simulink model "wushuadianji"  (R2020a)
settings: Solver=FixedStepAuto  StartTime=0.0  StopTime=Inf  FixedStep=Ts  RelTol=1e-3  EnableMultiTasking=on
model workspace (MAT data in the model file):
  Ts = 0.001
libraries: canmsglib x8, speedgoatlib_IO602_4 x3, CanManageLib x3
settings Model: Creator=HIL  LastModifiedBy=HIL
settings SolverCC: ConcurrentTasks=on  AutoInsertRateTranBlk=on
settings DataIOCC: SaveFormat=StructureWithTime
settings OptimizationCC: BlockReduction=off  OptimizeBlockIOStorage=off
settings HardwareCC: ProdBitPerPointer=32  ProdBitPerSizeT=32  ProdBitPerPtrDiffT=32  ProdLargestAtomicFloat=None  ProdWordSize=32  ProdLongLongMode=on  ProdHWDeviceType=Generic->32-bit x86 compatible
settings RTWCC: Description=Simulink Real-Time  SystemTargetFile=slrt.tlc  TemplateMakefile=slrt_default_tmf  CodeExecutionProfiling=on  RTWCompilerOptimization=on
settings SimulinkRealTimeCC: SupportVariableSizeSignals=on  RL32LogTETModifier=off  xPCConcurrentTasks=on

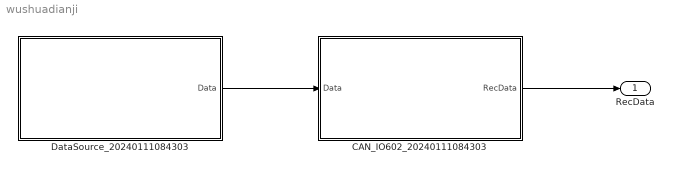
== system wushuadianji ==
  CAN_IO602_20240111084303 : Subsystem
  DataSource_20240111084303 : Subsystem
  RecData : Outport
  wires:
  DataSource_20240111084303/1(Data) -> CAN_IO602_20240111084303/1(Data)
  CAN_IO602_20240111084303/1(RecData) -> RecData/1

== system wushuadianji/CAN_IO602_20240111084303 ==
  Data : Inport
  CAN Receive : Subsystem  TreatAsAtomicUnit=on
  CAN Setup : speedgoatlib_IO602_4/Legacy/CAN Setup   moduletype=IO602  id=1  pciSlot=-1  chn1=CAN (HS)  chn2=CAN (HS)  chn3=Disabled  chn4=Disabled  initStruct=[]  termStruct=[]  ArbitrationbdrChn1=500 kBaud  ArbitrationManbdrChn1=[2,16,63,16]  FdbdrChn1=5.0 MBaud  FdManbdrChn1=[2,2,5,2]  ArbitrationbdrChn2=500 kBaud  ArbitrationManbdrChn2=[2,16,63,16]  FdbdrChn2=5.0 MBaud  FdManbdrChn2=[2,2,5,2]  ArbitrationbdrChn3=1.0 MBaud  ArbitrationManbdrChn3=[2,8,31,8]  FdbdrChn3=5.0 MBaud  FdManbdrChn3=[2,2,5,2]  ArbitrationbdrChn4=1.0 MBaud  ArbitrationManbdrChn4=[2,8,31,8]  FdbdrChn4=5.0 MBaud  FdManbdrChn4=[2,2,5,2]  moduleInitValues=[602 1 -1 -1]
      settings: SourceProductName=Simulink Real-Time: Speedgoat I/O Blockset
  CAN Transmit : Subsystem  TreatAsAtomicUnit=on
  Enable : BusSelector  OutputSignals=Trigger.Enable_CanTransmit
  RecData : Outport
  wires:
  Enable/1 -> CAN Transmit/Enable  "<Enable_CanTransmit>"
  Data/1 -> CAN Transmit/1(Data), Enable/1
  CAN Receive/1(RecData) -> RecData/1

== system wushuadianji/DataSource_20240111084303 ==
  Bus Creator : BusCreator  Inputs=2
  Signal : Subsystem
  Trigger : Subsystem
  Data : Outport
  wires:
  Trigger/1(Trigger) -> Bus Creator/1  "Trigger"
  Signal/1(Signal) -> Bus Creator/2  "Signal"
  Bus Creator/1 -> Data/1  "Data"

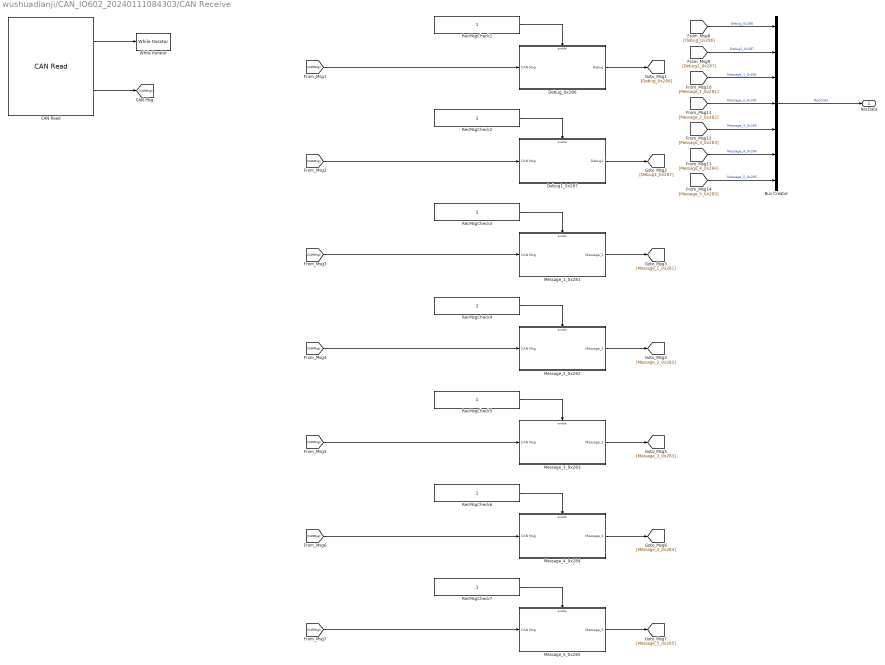
== system wushuadianji/CAN_IO602_20240111084303/CAN Receive ==
  Bus Creator : BusCreator  Inputs=7
  CAN Read : speedgoatlib_IO602_4/Legacy/CAN Read  id=1  ts=-1  channel=1  messageType=CAN  canType=CAN (HS)  BusOutput=on  initValues=[602 1 -1 0 1 1 1]
      settings: SourceProductName=Simulink Real-Time: Speedgoat I/O Blockset
  Debug1_0x287 : Subsystem  TreatAsAtomicUnit=on
  Debug_0x286 : Subsystem  TreatAsAtomicUnit=on
  Message_1_0x281 : Subsystem  TreatAsAtomicUnit=on
  Message_2_0x282 : Subsystem  TreatAsAtomicUnit=on
  Message_3_0x283 : Subsystem  TreatAsAtomicUnit=on
  Message_4_0x284 : Subsystem  TreatAsAtomicUnit=on
  Message_5_0x285 : Subsystem  TreatAsAtomicUnit=on
  RecMsgCheck{1..7} (7 alike) : Constant  OutDataTypeStr=boolean
  While Iterator : WhileIterator  MaxIters=500  WhileBlockType=do-while
  RecData : Outport
  wires:
  CAN Read/1 -> While Iterator/1
  CAN Read/2 -> [CANMsg]
  RecMsgCheck1/1 -> Debug_0x286/Enable
  [CANMsg] -> Debug_0x286/1(CAN Msg)
  Debug_0x286/1(Debug) -> [Debug_0x286]
  RecMsgCheck2/1 -> Debug1_0x287/Enable
  [CANMsg] -> Debug1_0x287/1(CAN Msg)
  Debug1_0x287/1(Debug1) -> [Debug1_0x287]
  RecMsgCheck3/1 -> Message_1_0x281/Enable
  [CANMsg] -> Message_1_0x281/1(CAN Msg)
  Message_1_0x281/1(Message_1) -> [Message_1_0x281]
  RecMsgCheck4/1 -> Message_2_0x282/Enable
  [CANMsg] -> Message_2_0x282/1(CAN Msg)
  Message_2_0x282/1(Message_2) -> [Message_2_0x282]
  RecMsgCheck5/1 -> Message_3_0x283/Enable
  [CANMsg] -> Message_3_0x283/1(CAN Msg)
  Message_3_0x283/1(Message_3) -> [Message_3_0x283]
  RecMsgCheck6/1 -> Message_4_0x284/Enable
  [CANMsg] -> Message_4_0x284/1(CAN Msg)
  Message_4_0x284/1(Message_4) -> [Message_4_0x284]
  RecMsgCheck7/1 -> Message_5_0x285/Enable
  [CANMsg] -> Message_5_0x285/1(CAN Msg)
  Message_5_0x285/1(Message_5) -> [Message_5_0x285]
  [Debug_0x286] -> Bus Creator/1  "Debug_0x286"
  [Debug1_0x287] -> Bus Creator/2  "Debug1_0x287"
  [Message_1_0x281] -> Bus Creator/3  "Message_1_0x281"
  [Message_2_0x282] -> Bus Creator/4  "Message_2_0x282"
  [Message_3_0x283] -> Bus Creator/5  "Message_3_0x283"
  [Message_4_0x284] -> Bus Creator/6  "Message_4_0x284"
  [Message_5_0x285] -> Bus Creator/7  "Message_5_0x285"
  Bus Creator/1 -> RecData/1  "RecData"

== system wushuadianji/CAN_IO602_20240111084303/CAN Transmit ==
  Data : Inport
  Enable : EnablePort
  Data1 : BusSelector  OutputSignals=Trigger.Vector__XXX,Signal.Vector__XXX
  Enable1 : BusSelector  OutputSignals=Enable_Vector__XXX
  Vector__XXX : Subsystem  TreatAsAtomicUnit=on
  wires:
  Data/1 -> Data1/1
  Data1/1 -> Vector__XXX/1(Trigger), Enable1/1  "<Vector__XXX>"
  Data1/2 -> Vector__XXX/2(Vector__XXX)  "<Vector__XXX>"
  Enable1/1 -> Vector__XXX/Enable  "<Enable_Vector__XXX>"

== system wushuadianji/DataSource_20240111084303/Signal ==
  Bus Creator : BusCreator  Inputs=1
  Signal_Vector__XXX : Subsystem
  Signal : Outport
  wires:
  Signal_Vector__XXX/1(Vector__XXX) -> Bus Creator/1  "Vector__XXX"
  Bus Creator/1 -> Signal/1  "Signal"

== system wushuadianji/DataSource_20240111084303/Trigger ==
  Bus Creator : BusCreator  Inputs=2
  Enable_CanTransmit : Constant
  Trigger_Vector__XXX : Subsystem
  Trigger : Outport
  wires:
  Trigger_Vector__XXX/1(Vector__XXX) -> Bus Creator/1  "Vector__XXX"
  Enable_CanTransmit/1 -> Bus Creator/2  "Enable_CanTransmit"
  Bus Creator/1 -> Trigger/1  "Trigger"

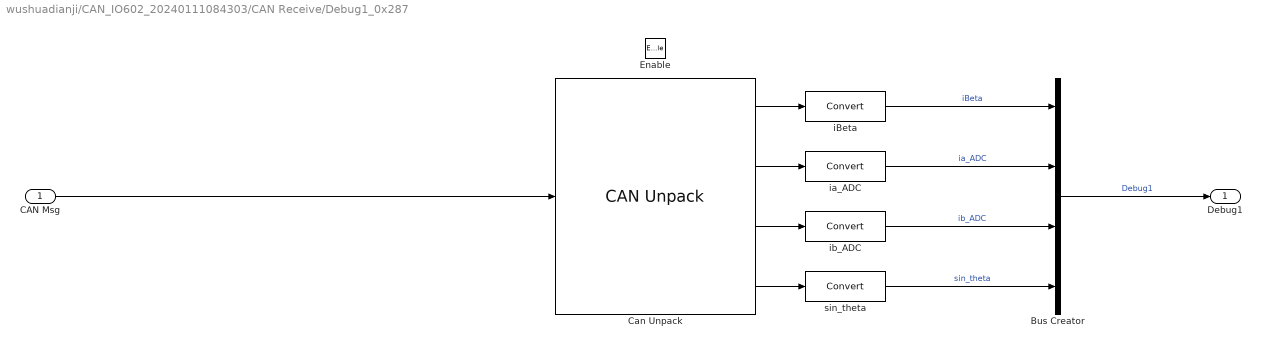
== system wushuadianji/CAN_IO602_20240111084303/CAN Receive/Debug1_0x287 ==
  CAN Msg : Inport
  Enable : EnablePort
  Bus Creator : BusCreator  Inputs=4
  Can Unpack : canmsglib/CAN Unpack  CANdbFile=F:\湖大艾盛\wushuadianji_20230612.dbc  MsgList=Debug1  MsgName=Debug1  MsgIDType=Standard (11-bit identifier)  MsgIdentifier=647  MsgLength=8  SignalInfo={'iBeta','8','16','BE','signed','Standard','0','0.01','0','-Inf','Inf';'ia_ADC','40','16','BE','unsigned','Standard','0','1','0','-Inf','Inf';'ib_ADC','56','16','BE','unsigned','Standard','0','1','0','-Inf','Inf';'sin_theta','24','16','BE','signed','Standard','0','0.001','0','-Inf','Inf'}  IDPort=off  TimestampPort=off  ErrorPort=off  RemotePort=off  LengthPort=off  StatusPort=off  ApplyMinMax=off
      settings: SourceProductBaseCode=ME,VN  DataFormat=CANdb specified signals
  iBeta : DataTypeConversion
  ia_ADC : DataTypeConversion
  ib_ADC : DataTypeConversion
  sin_theta : DataTypeConversion
  Debug1 : Outport
  wires:
  CAN Msg/1 -> Can Unpack/1
  Can Unpack/1 -> iBeta/1
  iBeta/1 -> Bus Creator/1  "iBeta"
  Can Unpack/2 -> ia_ADC/1
  ia_ADC/1 -> Bus Creator/2  "ia_ADC"
  Can Unpack/3 -> ib_ADC/1
  ib_ADC/1 -> Bus Creator/3  "ib_ADC"
  Can Unpack/4 -> sin_theta/1
  sin_theta/1 -> Bus Creator/4  "sin_theta"
  Bus Creator/1 -> Debug1/1  "Debug1"

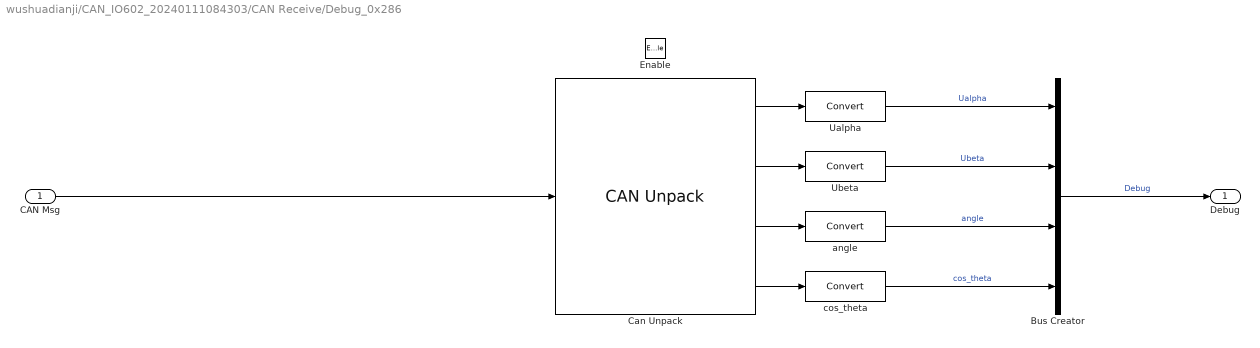
== system wushuadianji/CAN_IO602_20240111084303/CAN Receive/Debug_0x286 ==
  CAN Msg : Inport
  Enable : EnablePort
  Bus Creator : BusCreator  Inputs=4
  Can Unpack : canmsglib/CAN Unpack  CANdbFile=F:\湖大艾盛\wushuadianji_20230612.dbc  MsgList=Debug  MsgName=Debug  MsgIDType=Standard (11-bit identifier)  MsgIdentifier=646  MsgLength=8  SignalInfo={'Ualpha','40','16','BE','signed','Standard','0','1','0','-Inf','Inf';'Ubeta','56','16','BE','signed','Standard','0','1','0','-Inf','Inf';'angle','8','16','BE','unsigned','Standard','0','1','0','-Inf','Inf';'cos_theta','24','16','BE','signed','Standard','0','0.001','0','-Inf','Inf'}  IDPort=off  TimestampPort=off  ErrorPort=off  RemotePort=off  LengthPort=off  StatusPort=off  ApplyMinMax=off
      settings: SourceProductBaseCode=ME,VN  DataFormat=CANdb specified signals
  Ualpha : DataTypeConversion
  Ubeta : DataTypeConversion
  angle : DataTypeConversion
  cos_theta : DataTypeConversion
  Debug : Outport
  wires:
  CAN Msg/1 -> Can Unpack/1
  Can Unpack/1 -> Ualpha/1
  Ualpha/1 -> Bus Creator/1  "Ualpha"
  Can Unpack/2 -> Ubeta/1
  Ubeta/1 -> Bus Creator/2  "Ubeta"
  Can Unpack/3 -> angle/1
  angle/1 -> Bus Creator/3  "angle"
  Can Unpack/4 -> cos_theta/1
  cos_theta/1 -> Bus Creator/4  "cos_theta"
  Bus Creator/1 -> Debug/1  "Debug"

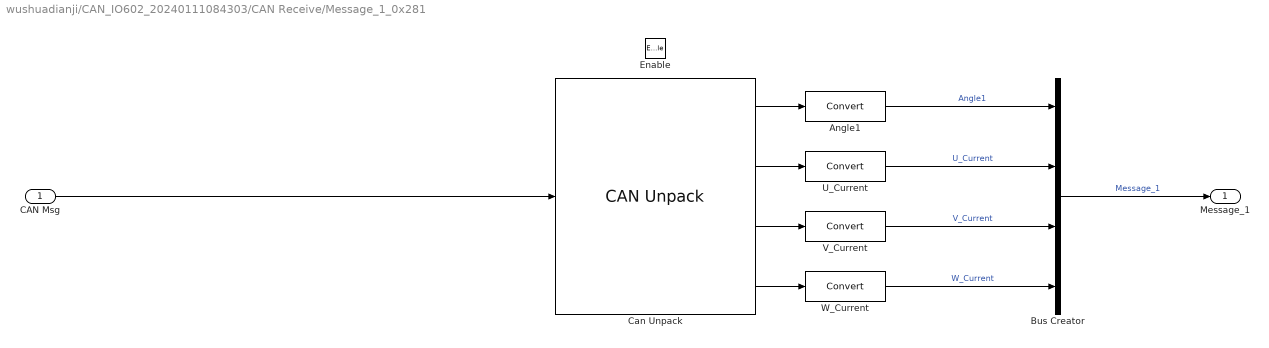
== system wushuadianji/CAN_IO602_20240111084303/CAN Receive/Message_1_0x281 ==
  CAN Msg : Inport
  Enable : EnablePort
  Angle1 : DataTypeConversion
  Bus Creator : BusCreator  Inputs=4
  Can Unpack : canmsglib/CAN Unpack  CANdbFile=F:\湖大艾盛\wushuadianji_20230612.dbc  MsgList=Message_1  MsgName=Message_1  MsgIDType=Standard (11-bit identifier)  MsgIdentifier=641  MsgLength=8  SignalInfo={'Angle1','56','16','BE','signed','Standard','0','1','0','-Inf','Inf';'U_Current','8','16','BE','signed','Standard','0','1','0','-Inf','Inf';'V_Current','24','16','BE','signed','Standard','0','1','0','-Inf','Inf';'W_Current','40','16','BE','signed','Standard','0','1','0','-Inf','Inf'}  IDPort=off  TimestampPort=off  ErrorPort=off  RemotePort=off  LengthPort=off  StatusPort=off  ApplyMinMax=off
      settings: SourceProductBaseCode=ME,VN  DataFormat=CANdb specified signals
  U_Current : DataTypeConversion
  V_Current : DataTypeConversion
  W_Current : DataTypeConversion
  Message_1 : Outport
  wires:
  CAN Msg/1 -> Can Unpack/1
  Can Unpack/1 -> Angle1/1
  Angle1/1 -> Bus Creator/1  "Angle1"
  Can Unpack/2 -> U_Current/1
  U_Current/1 -> Bus Creator/2  "U_Current"
  Can Unpack/3 -> V_Current/1
  V_Current/1 -> Bus Creator/3  "V_Current"
  Can Unpack/4 -> W_Current/1
  W_Current/1 -> Bus Creator/4  "W_Current"
  Bus Creator/1 -> Message_1/1  "Message_1"

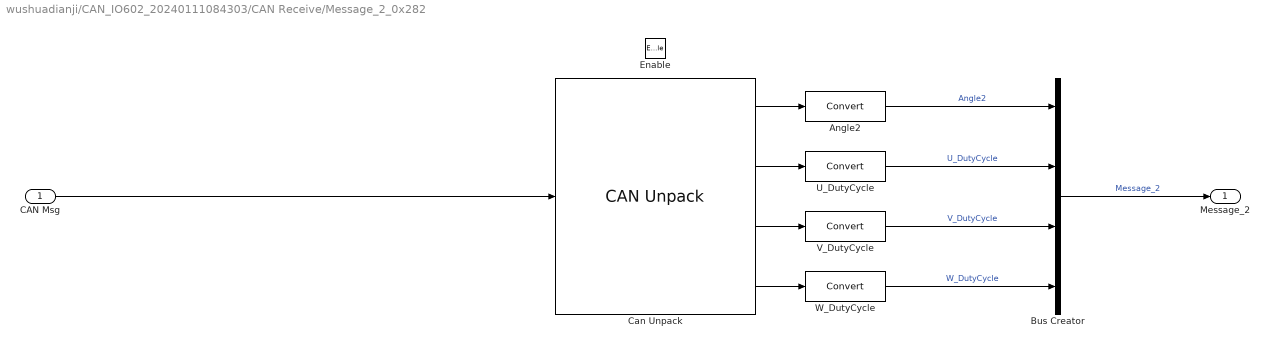
== system wushuadianji/CAN_IO602_20240111084303/CAN Receive/Message_2_0x282 ==
  CAN Msg : Inport
  Enable : EnablePort
  Angle2 : DataTypeConversion
  Bus Creator : BusCreator  Inputs=4
  Can Unpack : canmsglib/CAN Unpack  CANdbFile=F:\湖大艾盛\wushuadianji_20230612.dbc  MsgList=Message_2  MsgName=Message_2  MsgIDType=Standard (11-bit identifier)  MsgIdentifier=642  MsgLength=8  SignalInfo={'Angle2','8','16','BE','signed','Standard','0','1','0','-Inf','Inf';'U_DutyCycle','24','16','BE','signed','Standard','0','1','0','-Inf','Inf';'V_DutyCycle','40','16','BE','signed','Standard','0','1','0','-Inf','Inf';'W_DutyCycle','56','16','BE','signed','Standard','0','1','0','-Inf','Inf'}  IDPort=off  TimestampPort=off  ErrorPort=off  RemotePort=off  LengthPort=off  StatusPort=off  ApplyMinMax=off
      settings: SourceProductBaseCode=ME,VN  DataFormat=CANdb specified signals
  U_DutyCycle : DataTypeConversion
  V_DutyCycle : DataTypeConversion
  W_DutyCycle : DataTypeConversion
  Message_2 : Outport
  wires:
  CAN Msg/1 -> Can Unpack/1
  Can Unpack/1 -> Angle2/1
  Angle2/1 -> Bus Creator/1  "Angle2"
  Can Unpack/2 -> U_DutyCycle/1
  U_DutyCycle/1 -> Bus Creator/2  "U_DutyCycle"
  Can Unpack/3 -> V_DutyCycle/1
  V_DutyCycle/1 -> Bus Creator/3  "V_DutyCycle"
  Can Unpack/4 -> W_DutyCycle/1
  W_DutyCycle/1 -> Bus Creator/4  "W_DutyCycle"
  Bus Creator/1 -> Message_2/1  "Message_2"

== system wushuadianji/CAN_IO602_20240111084303/CAN Receive/Message_3_0x283 ==
  CAN Msg : Inport
  Enable : EnablePort
  Bus Creator : BusCreator  Inputs=2
  Can Unpack : canmsglib/CAN Unpack  CANdbFile=F:\湖大艾盛\wushuadianji_20230612.dbc  MsgList=Message_3  MsgName=Message_3  MsgIDType=Standard (11-bit identifier)  MsgIdentifier=643  MsgLength=8  SignalInfo={'ia_act','24','32','BE','signed','Standard','0','1','0','-Inf','Inf';'ib_act','56','32','BE','signed','Standard','0','1','0','-Inf','Inf'}  IDPort=off  TimestampPort=off  ErrorPort=off  RemotePort=off  LengthPort=off  StatusPort=off  ApplyMinMax=off
      settings: SourceProductBaseCode=ME,VN  DataFormat=CANdb specified signals
  ia_act : DataTypeConversion
  ib_act : DataTypeConversion
  Message_3 : Outport
  wires:
  CAN Msg/1 -> Can Unpack/1
  Can Unpack/1 -> ia_act/1
  ia_act/1 -> Bus Creator/1  "ia_act"
  Can Unpack/2 -> ib_act/1
  ib_act/1 -> Bus Creator/2  "ib_act"
  Bus Creator/1 -> Message_3/1  "Message_3"

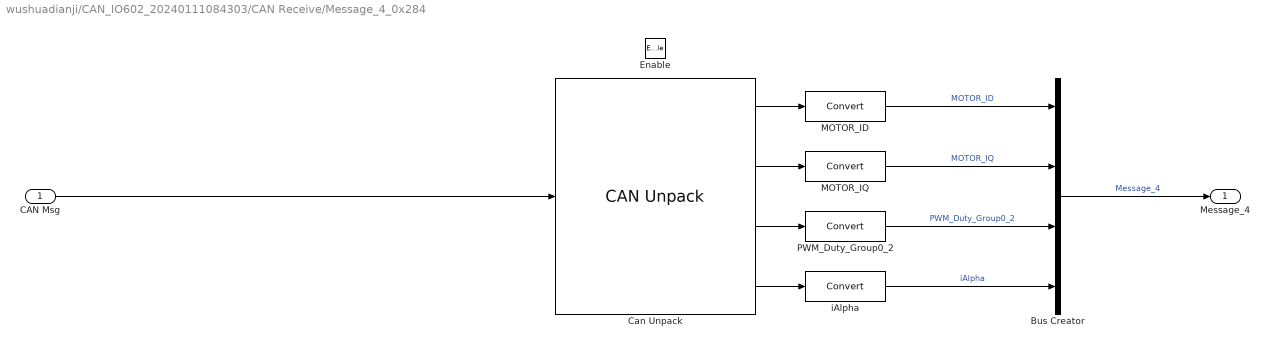
== system wushuadianji/CAN_IO602_20240111084303/CAN Receive/Message_4_0x284 ==
  CAN Msg : Inport
  Enable : EnablePort
  Bus Creator : BusCreator  Inputs=4
  Can Unpack : canmsglib/CAN Unpack  CANdbFile=F:\湖大艾盛\wushuadianji_20230612.dbc  MsgList=Message_4  MsgName=Message_4  MsgIDType=Standard (11-bit identifier)  MsgIdentifier=644  MsgLength=8  SignalInfo={'MOTOR_ID','24','16','BE','signed','Standard','0','0.01','0','-Inf','Inf';'MOTOR_IQ','40','16','BE','signed','Standard','0','0.01','0','-Inf','Inf';'PWM_Duty_Group0_2','8','16','BE','unsigned','Standard','0','0.013333','0','-Inf','Inf';'iAlpha','56','16','BE','signed','Standard','0','0.01','0','-Inf','Inf'}  IDPort=off  TimestampPort=off  ErrorPort=off  RemotePort=off  LengthPort=off  StatusPort=off  ApplyMinMax=off
      settings: SourceProductBaseCode=ME,VN  DataFormat=CANdb specified signals
  MOTOR_ID : DataTypeConversion
  MOTOR_IQ : DataTypeConversion
  PWM_Duty_Group0_2 : DataTypeConversion
  iAlpha : DataTypeConversion
  Message_4 : Outport
  wires:
  CAN Msg/1 -> Can Unpack/1
  Can Unpack/1 -> MOTOR_ID/1
  MOTOR_ID/1 -> Bus Creator/1  "MOTOR_ID"
  Can Unpack/2 -> MOTOR_IQ/1
  MOTOR_IQ/1 -> Bus Creator/2  "MOTOR_IQ"
  Can Unpack/3 -> PWM_Duty_Group0_2/1
  PWM_Duty_Group0_2/1 -> Bus Creator/3  "PWM_Duty_Group0_2"
  Can Unpack/4 -> iAlpha/1
  iAlpha/1 -> Bus Creator/4  "iAlpha"
  Bus Creator/1 -> Message_4/1  "Message_4"

== system wushuadianji/CAN_IO602_20240111084303/CAN Receive/Message_5_0x285 ==
  CAN Msg : Inport
  Enable : EnablePort
  Bus Creator : BusCreator  Inputs=3
  Can Unpack : canmsglib/CAN Unpack  CANdbFile=F:\湖大艾盛\wushuadianji_20230612.dbc  MsgList=Message_5  MsgName=Message_5  MsgIDType=Standard (11-bit identifier)  MsgIdentifier=645  MsgLength=8  SignalInfo={'PWM_Duty_Group0_0','40','16','BE','unsigned','Standard','0','0.013333','0','-Inf','Inf';'PWM_Duty_Group0_1','56','16','BE','unsigned','Standard','0','0.013333','0','0','873.8';'veelspeed','24','32','BE','signed','Standard','0','0.16667','0','-Inf','Inf'}  IDPort=off  TimestampPort=off  ErrorPort=off  RemotePort=off  LengthPort=off  StatusPort=off  ApplyMinMax=off
      settings: SourceProductBaseCode=ME,VN  DataFormat=CANdb specified signals
  PWM_Duty_Group0_0 : DataTypeConversion
  PWM_Duty_Group0_1 : DataTypeConversion
  veelspeed : DataTypeConversion
  Message_5 : Outport
  wires:
  CAN Msg/1 -> Can Unpack/1
  Can Unpack/1 -> PWM_Duty_Group0_0/1
  PWM_Duty_Group0_0/1 -> Bus Creator/1  "PWM_Duty_Group0_0"
  Can Unpack/2 -> PWM_Duty_Group0_1/1
  PWM_Duty_Group0_1/1 -> Bus Creator/2  "PWM_Duty_Group0_1"
  Can Unpack/3 -> veelspeed/1
  veelspeed/1 -> Bus Creator/3  "veelspeed"
  Bus Creator/1 -> Message_5/1  "Message_5"

== system wushuadianji/CAN_IO602_20240111084303/CAN Transmit/Vector__XXX ==
  Trigger : Inport
  Vector__XXX : Inport  Port=2
  Enable : EnablePort
  Bus Selector : BusSelector  OutputSignals=Trigger_VCU_BrakingRequest_0x120,Enable_VCU_BrakingRequest_0x120
  Bus Selector1 : BusSelector  OutputSignals=VCU_BrakingRequest_0x120
  VCU_BrakingRequest_0x120 : Subsystem  TreatAsAtomicUnit=on
  wires:
  Trigger/1 -> Bus Selector/1
  Bus Selector/1 -> VCU_BrakingRequest_0x120/Trigger  "<Trigger_VCU_BrakingRequest_0x120>"
  Bus Selector/2 -> VCU_BrakingRequest_0x120/Enable  "<Enable_VCU_BrakingRequest_0x120>"
  Bus Selector1/1 -> VCU_BrakingRequest_0x120/1(VCU_BrakingRequest)  "<VCU_BrakingRequest_0x120>"
  Vector__XXX/1 -> Bus Selector1/1

== system wushuadianji/DataSource_20240111084303/Signal/Signal_Vector__XXX ==
  Bus Creator : BusCreator  Inputs=1
  VCU_BrakingRequest_0x120 : Subsystem
  Vector__XXX : Outport
  wires:
  VCU_BrakingRequest_0x120/1(VCU_BrakingRequest_0x120) -> Bus Creator/1  "VCU_BrakingRequest_0x120"
  Bus Creator/1 -> Vector__XXX/1  "Vector__XXX"

== system wushuadianji/DataSource_20240111084303/Trigger/Trigger_Vector__XXX ==
  Bus Creator : BusCreator  Inputs=3
  Enable_VCU_BrakingRequest_0x120 : Constant
  Enable_Vector__XXX : Constant
  Trigger_VCU_BrakingRequest_0x120 : Subsystem  mask(Cansend trigger mode selection){ModeSelect=1, EnablePeriod=0.001, Period=50, MsgLstCnt=0}
      mask prompts: EnablePeriod "EnablePeriod(s)"; Period "Period(ms)"
      mask help:
      | ModeSelect value description :
      | 1:period of transmission
      | 2: manually send
      | 3:conditional trigger
      mask TypeOptions ModeSelect: 1 | 2 | 3
      mask Callback ModeSelect:
      | mode = get(gcbh,'ModeSelect');
      | 
      | if(mode == '3')
      |     if(isempty(find_system(gcb,'LookUnderMasks','on','SearchDepth',1,'BlockType','Inport')))
      |         path = get(gcbh,'Path');
      |         name = get(gcbh,'Name');
      |         find_system(gcbh,'block','');
      |         inportsource  = 'simulink/Sources/In1';
      |         inportdist = [path,'/',name,'/','ConditionalTrigger'];
      |         handle_tmp = find_system(gcbh,'name','ConditionalTrigger');
      |         position_tmp = get_param(inportdist,'Position');
      | 
      |         delete_block(inportdist);
      |         add_block(inportsource,inportdist,'Position',position_tmp);
      | 
      |     else
      | 
      |     end
      | else
      |     path = get(gcbh,'Path');
      |     name = get(gcbh,'Name');
      |     find_system(gcbh,'block','');
      |     inportsource  = 'simulink/Sources/Ground';
      |     inportdist = [path,'/',name,'/','ConditionalTrigger'];
      |     handle_tmp = find_system(gcbh,'name','ConditionalTrigger');
      |     position_tmp = get_param(inportdist,'Position');
      | 
      |     delete_block(inportdist);
      |     add_block(inportsource,inportdist,'Position',position_tmp);
      | 
      | 
      | end
      mask Display:
      | plot([0 0.3 0.3 0.7 0.7 1],[0.1 0.1 0.8 0.8 0.1 0.1]);
      | port_label('output', 1, 'CndTriggerout');
      | if(isempty(find_system(gcb,'LookUnderMasks','on','SearchDepth',1,'BlockType','Inport')))
      | else
      |    port_label('input', 1, 'CndTriggerin');
      | end
  Vector__XXX : Outport
  wires:
  Enable_VCU_BrakingRequest_0x120/1 -> Bus Creator/1  "Enable_VCU_BrakingRequest_0x120"
  Trigger_VCU_BrakingRequest_0x120/1(Out1) -> Bus Creator/2  "Trigger_VCU_BrakingRequest_0x120"
  Enable_Vector__XXX/1 -> Bus Creator/3  "Enable_Vector__XXX"
  Bus Creator/1 -> Vector__XXX/1  "Vector__XXX"

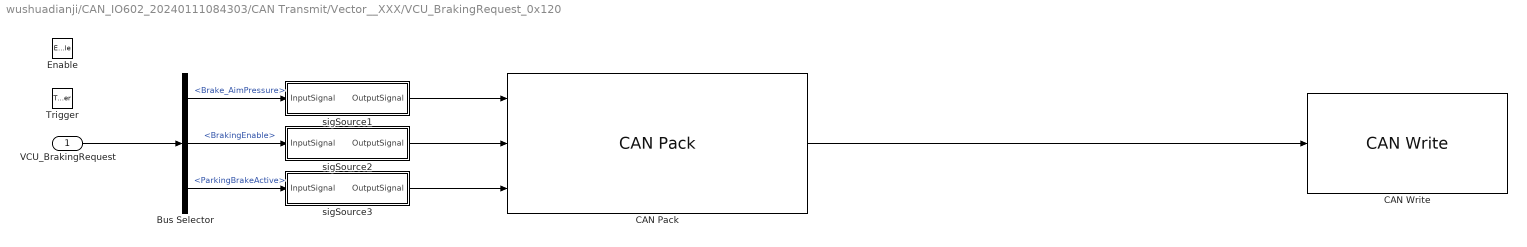
== system wushuadianji/CAN_IO602_20240111084303/CAN Transmit/Vector__XXX/VCU_BrakingRequest_0x120 ==
  VCU_BrakingRequest : Inport
  Enable : EnablePort
  Trigger : TriggerPort  VariantControl=Variant
  Bus Selector : BusSelector  OutputSignals=Brake_AimPressure,BrakingEnable,ParkingBrakeActive
  CAN Pack : canmsglib/CAN Pack  CANdbFile=F:\湖大艾盛\wushuadianji_20230612.dbc  MsgList=VCU_BrakingRequest  MsgName=VCU_BrakingRequest  MsgIDType=Standard (11-bit identifier)  MsgIdentifier=288  MsgLength=8  Remote=off  ApplyMinMax=off  BusOutput=on  SignalInfo={'Brake_AimPressure','8','8','BE','unsigned','Standard','0','0.1','0','-Inf','Inf';'BrakingEnable','0','4','BE','unsigned','Standard','0','1','0','-Inf','Inf';'ParkingBrakeActive','4','4','BE','unsigned','Standard','0','1','0','-Inf','Inf'}
      settings: SourceProductBaseCode=ME,VN  DataFormat=CANdb specified signals
  CAN Write : speedgoatlib_IO602_4/Legacy/CAN Write  id=1  ts=-1  channel=1  messageType=CAN  BusInput=on  enableStatusPort=off  canType=CAN (HS)  initValues=[602 1 -1 0 1 1 0 1]
      settings: SourceProductName=Simulink Real-Time: Speedgoat I/O Blockset
  sigSource1 : Subsystem
  sigSource2 : Subsystem
  sigSource3 : Subsystem
  wires:
  VCU_BrakingRequest/1 -> Bus Selector/1
  Bus Selector/1 -> sigSource1/1(InputSignal)  "<Brake_AimPressure>"
  sigSource1/1(OutputSignal) -> CAN Pack/1
  Bus Selector/2 -> sigSource2/1(InputSignal)  "<BrakingEnable>"
  sigSource2/1(OutputSignal) -> CAN Pack/2
  Bus Selector/3 -> sigSource3/1(InputSignal)  "<ParkingBrakeActive>"
  sigSource3/1(OutputSignal) -> CAN Pack/3
  CAN Pack/1 -> CAN Write/1

== system wushuadianji/DataSource_20240111084303/Signal/Signal_Vector__XXX/VCU_BrakingRequest_0x120 ==
  Brake_AimPressure : Constant  Value=0
  BrakingEnable : Constant  Value=0
  Bus Creator : BusCreator  Inputs=3
  ParkingBrakeActive : Constant  Value=0
  dtc1 : DataTypeConversion
  dtc2 : DataTypeConversion
  dtc3 : DataTypeConversion
  VCU_BrakingRequest_0x120 : Outport
  wires:
  dtc1/1 -> Bus Creator/1  "Brake_AimPressure"
  Brake_AimPressure/1 -> dtc1/1  "Brake_AimPressure"
  dtc2/1 -> Bus Creator/2  "BrakingEnable"
  BrakingEnable/1 -> dtc2/1  "BrakingEnable"
  dtc3/1 -> Bus Creator/3  "ParkingBrakeActive"
  ParkingBrakeActive/1 -> dtc3/1  "ParkingBrakeActive"
  Bus Creator/1 -> VCU_BrakingRequest_0x120/1  "VCU_BrakingRequest_0x120"

== system wushuadianji/DataSource_20240111084303/Trigger/Trigger_Vector__XXX/Trigger_VCU_BrakingRequest_0x120 ==
  note: 发送触发方式的拓展：
      | 1、循环周期发送(包括丢帧方式)；
      | 2、手动触发发送(增加调试模块)；
      | 3、待拓展模式；
  ConditionalTrigger : Ground
  Cycle : Subsystem
  Kick : Subsystem
  KickValueChange : Subsystem
      settings: OpenFcn=|
      | KickValuePath =[gcs,'/Kick/KickValue'];
      | KickValueTmp = str2num(get_param(KickValuePath,'Value'));
      | if KickValueTmp == 1
      | set_param(KickValuePath,'Value','0');
      | else
      | set_param(KickValuePath,'Value','1');
      | end
      | masKicks = Simulink.Mask.get(gcb);
      | DispKicks = sprintf('disp("KicksValue:%s")',get_param(KickValuePath,'Value'));
      | masKicks.Display = DispKicks;
      mask Display: disp("KicksValue:1")
  ModeSelect : Constant  Value=ModeSelect  SampleTime=-1
  Multiport Switch : MultiPortSwitch
  Out1 : Outport  VectorParamsAs1DForOutWhenUnconnected=off
  wires:
  ConditionalTrigger/1 -> Multiport Switch/4
  Multiport Switch/1 -> Out1/1
  ModeSelect/1 -> Multiport Switch/1
  Cycle/1(Out1) -> Multiport Switch/2
  Kick/1(Out1) -> Multiport Switch/3

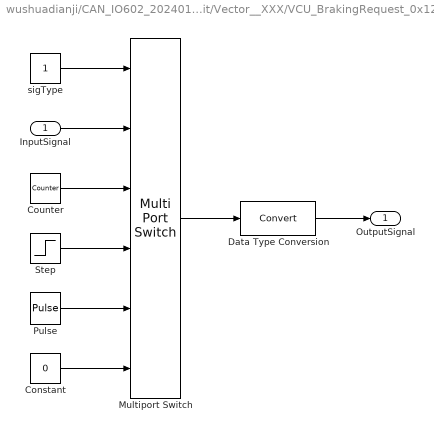
== system wushuadianji/CAN_IO602_20240111084303/CAN Transmit/Vector__XXX/VCU_BrakingRequest_0x120/sigSource1 ==
  InputSignal : Inport
  Constant : Constant  Value=0
  Counter : CanManageLib/Counter  initValue=0  finalValue=15  stepValue=1
  Data Type Conversion : DataTypeConversion
  Multiport Switch : MultiPortSwitch  Inputs=5
  Pulse : DiscretePulseGenerator  Period=10  PulseWidth=5  SampleTime=-1
  Step : Step
  sigType : Constant
  OutputSignal : Outport
  wires:
  Data Type Conversion/1 -> OutputSignal/1
  Multiport Switch/1 -> Data Type Conversion/1
  Pulse/1 -> Multiport Switch/5
  Step/1 -> Multiport Switch/4
  Counter/1 -> Multiport Switch/3
  Constant/1 -> Multiport Switch/6
  InputSignal/1 -> Multiport Switch/2
  sigType/1 -> Multiport Switch/1

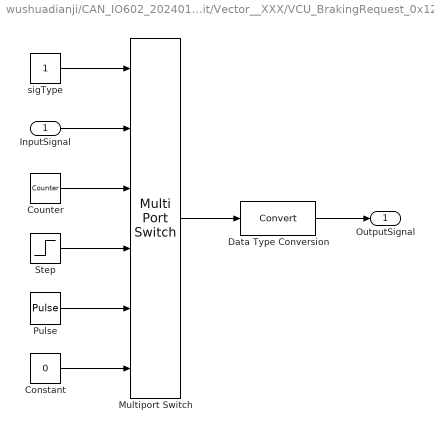
== system wushuadianji/CAN_IO602_20240111084303/CAN Transmit/Vector__XXX/VCU_BrakingRequest_0x120/sigSource2 ==
  InputSignal : Inport
  Constant : Constant  Value=0
  Counter : CanManageLib/Counter  initValue=0  finalValue=15  stepValue=1
  Data Type Conversion : DataTypeConversion
  Multiport Switch : MultiPortSwitch  Inputs=5
  Pulse : DiscretePulseGenerator  Period=10  PulseWidth=5  SampleTime=-1
  Step : Step
  sigType : Constant
  OutputSignal : Outport
  wires:
  Data Type Conversion/1 -> OutputSignal/1
  Multiport Switch/1 -> Data Type Conversion/1
  Pulse/1 -> Multiport Switch/5
  Step/1 -> Multiport Switch/4
  Counter/1 -> Multiport Switch/3
  Constant/1 -> Multiport Switch/6
  InputSignal/1 -> Multiport Switch/2
  sigType/1 -> Multiport Switch/1

== system wushuadianji/CAN_IO602_20240111084303/CAN Transmit/Vector__XXX/VCU_BrakingRequest_0x120/sigSource3 ==
  InputSignal : Inport
  Constant : Constant  Value=0
  Counter : CanManageLib/Counter  initValue=0  finalValue=15  stepValue=1
  Data Type Conversion : DataTypeConversion
  Multiport Switch : MultiPortSwitch  Inputs=5
  Pulse : DiscretePulseGenerator  Period=10  PulseWidth=5  SampleTime=-1
  Step : Step
  sigType : Constant
  OutputSignal : Outport
  wires:
  Data Type Conversion/1 -> OutputSignal/1
  Multiport Switch/1 -> Data Type Conversion/1
  Pulse/1 -> Multiport Switch/5
  Step/1 -> Multiport Switch/4
  Counter/1 -> Multiport Switch/3
  Constant/1 -> Multiport Switch/6
  InputSignal/1 -> Multiport Switch/2
  sigType/1 -> Multiport Switch/1

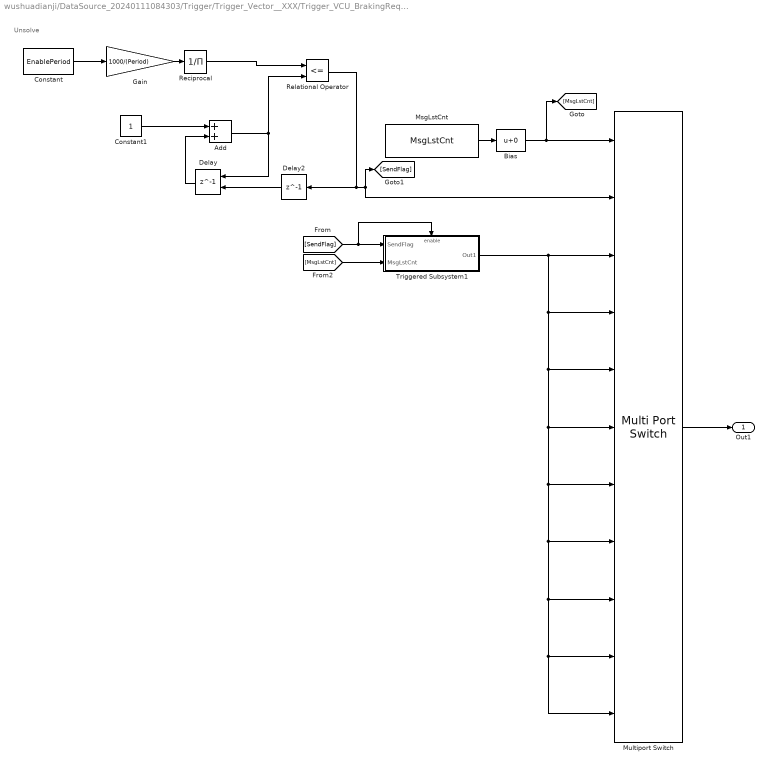
== system wushuadianji/DataSource_20240111084303/Trigger/Trigger_Vector__XXX/Trigger_VCU_BrakingRequest_0x120/Cycle ==
  note: Unsolve
  Add : Sum
  Bias : Bias
  Constant : Constant  Value=EnablePeriod  SampleTime=-1
  Constant1 : Constant  SampleTime=-1
  Delay : Delay  DelayLength=1  ExternalReset=Rising
      settings: InputPortMap=u0,r5
  Delay2 : Delay  DelayLength=1
  Gain : Gain  Gain=1000/(Period)
  MsgLstCnt : Constant  Value=MsgLstCnt  SampleTime=-1
  Multiport Switch : MultiPortSwitch  DataPortOrder=Zero-based contiguous  Inputs=9  DataPortForDefault=Additional data port  zeroidx=on
  Reciprocal : Product  Inputs=/
  Relational Operator : RelationalOperator  Operator=<=  OutDataTypeStr=boolean  RndMeth=Simplest
  Triggered Subsystem1 : Subsystem  TreatAsAtomicUnit=on
  Out1 : Outport  VectorParamsAs1DForOutWhenUnconnected=off
  wires:
  Reciprocal/1 -> Relational Operator/1
  Constant1/1 -> Add/1
  Constant/1 -> Gain/1
  Gain/1 -> Reciprocal/1
  Add/1 -> Relational Operator/2, Delay/1
  Relational Operator/1 -> [SendFlag], Multiport Switch/2, Delay2/1
  Delay/1 -> Add/2
  Delay2/1 -> Delay/2
  Multiport Switch/1 -> Out1/1
  MsgLstCnt/1 -> Bias/1
  Triggered Subsystem1/1(Out1) -> Multiport Switch/4, Multiport Switch/5, Multiport Switch/6, Multiport Switch/7, Multiport Switch/8, Multiport Switch/9, Multiport Switch/10, Multiport Switch/11, Multiport Switch/3
  [MsgLstCnt] -> Triggered Subsystem1/2(MsgLstCnt)
  [SendFlag] -> Triggered Subsystem1/Enable, Triggered Subsystem1/1(SendFlag)
  Bias/1 -> Multiport Switch/1, [MsgLstCnt]

== system wushuadianji/DataSource_20240111084303/Trigger/Trigger_Vector__XXX/Trigger_VCU_BrakingRequest_0x120/Kick ==
  Delay1 : Delay  DelayLength=1
  KickValue : Constant  SampleTime=-1
  Relational Operator1 : RelationalOperator  Operator=~=  OutDataTypeStr=boolean  RndMeth=Simplest
  Out1 : Outport  VectorParamsAs1DForOutWhenUnconnected=off
  wires:
  KickValue/1 -> Delay1/1, Relational Operator1/1
  Delay1/1 -> Relational Operator1/2
  Relational Operator1/1 -> Out1/1

== system wushuadianji/DataSource_20240111084303/Trigger/Trigger_Vector__XXX/Trigger_VCU_BrakingRequest_0x120/KickValueChange ==

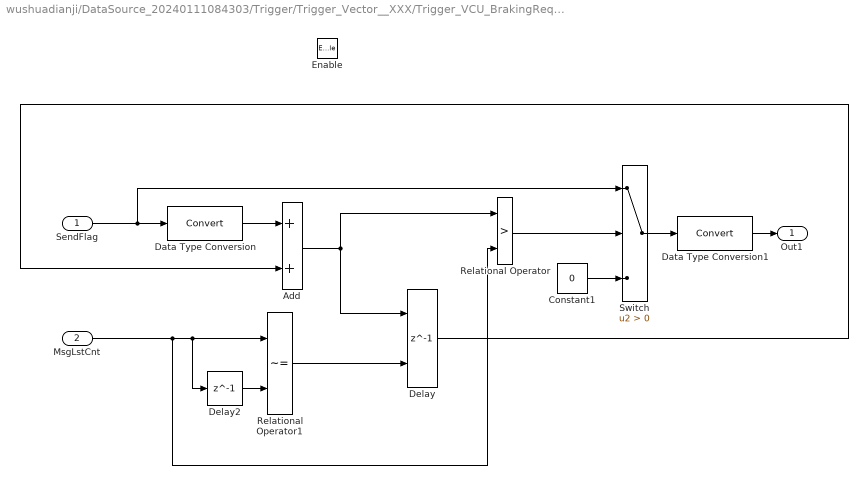
== system wushuadianji/DataSource_20240111084303/Trigger/Trigger_Vector__XXX/Trigger_VCU_BrakingRequest_0x120/Cycle/Triggered Subsystem1 ==
  SendFlag : Inport
  MsgLstCnt : Inport  Port=2
  Enable : EnablePort
  Add : Sum
  Constant1 : Constant  Value=0  SampleTime=-1
  Data Type Conversion : DataTypeConversion
  Data Type Conversion1 : DataTypeConversion
  Delay : Delay  DelayLength=1  ExternalReset=Rising
      settings: InputPortMap=u0,r5
  Delay2 : Delay  DelayLength=1
  Relational Operator : RelationalOperator  Operator=>  OutDataTypeStr=boolean  RndMeth=Simplest
  Relational Operator1 : RelationalOperator  Operator=~=  OutDataTypeStr=boolean  RndMeth=Simplest
  Switch : Switch  Criteria=u2 > Threshold
  Out1 : Outport  OutputWhenDisabled=reset  InitialOutput=0  VectorParamsAs1DForOutWhenUnconnected=off
  wires:
  Delay2/1 -> Relational Operator1/2
  Delay/1 -> Add/2
  Relational Operator1/1 -> Delay/2
  Data Type Conversion/1 -> Add/1
  Data Type Conversion1/1 -> Out1/1
  SendFlag/1 -> Data Type Conversion/1, Switch/1
  Constant1/1 -> Switch/3
  Switch/1 -> Data Type Conversion1/1
  Relational Operator/1 -> Switch/2
  MsgLstCnt/1 -> Relational Operator1/1, Delay2/1, Relational Operator/2
  Add/1 -> Relational Operator/1, Delay/1
